simulink model "Flatten2"  (Simulink 7.9)
settings: Solver=ode45  StartTime=0.0  StopTime=10.0  RelTol=1e-3
settings Model: Creator=boakes  LastModifiedBy=boakes

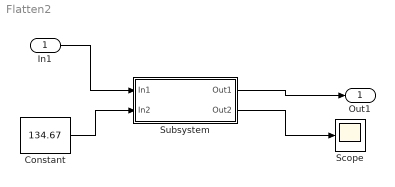
== system Flatten2 ==
  In1 : Inport
  Constant : Constant  Value=134.67
  Scope : Scope
  Subsystem : Subsystem
  Out1 : Outport
  wires:
  Subsystem/1(Out1) -> Out1/1
  Subsystem/2(Out2) -> Scope/1
  In1/1 -> Subsystem/1(In1)
  Constant/1 -> Subsystem/2(In2)

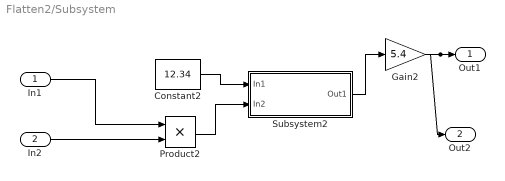
== system Flatten2/Subsystem ==
  In1 : Inport
  In2 : Inport  Port=2
  Constant2 : Constant  Value=12.34
  Gain2 : Gain  Gain=5.4
  Product2 : Product  RndMeth=Zero
  Subsystem2 : Subsystem
  Out1 : Outport
  Out2 : Outport  Port=2
  wires:
  In1/1 -> Product2/1
  In2/1 -> Product2/2
  Gain2/1 -> Out1/1, Out2/1
  Subsystem2/1(Out1) -> Gain2/1
  Product2/1 -> Subsystem2/2(In2)
  Constant2/1 -> Subsystem2/1(In1)

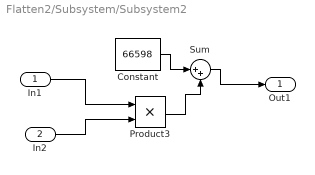
== system Flatten2/Subsystem/Subsystem2 ==
  In1 : Inport
  In2 : Inport  Port=2
  Constant : Constant  Value=66598
  Product3 : Product  RndMeth=Zero
  Sum : Sum  Inputs=|++
  Out1 : Outport
  wires:
  In1/1 -> Product3/1
  In2/1 -> Product3/2
  Product3/1 -> Sum/2
  Sum/1 -> Out1/1
  Constant/1 -> Sum/1
